simulink model "one_dim_sim"  (R2023a)
settings: Solver=VariableStepAuto  StartTime=0.0  StopTime=140  RelTol=1e-3
undefined symbols (not defined in the file): area_f, cd, g, mass, rho_m, volume
settings Model: Creator=erick  LastModifiedBy=erick

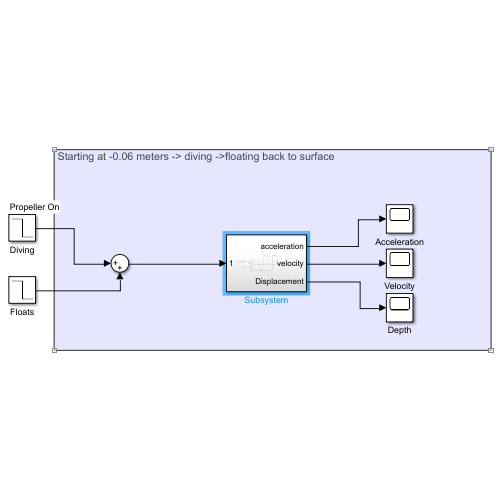
[thumbnail: Simulink's stored preview of the top-level diagram]
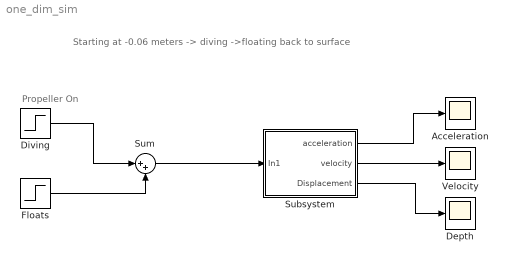
== system one_dim_sim ==
  note: Propeller On
  note: Starting at -0.06 meters -> diving ->floating back to surface
  Acceleration : Scope
  Depth : Scope
  Diving : Step  Time=60  Before=1.9  SampleTime=5
  Floats : Step  Time=80  After=-1  SampleTime=0
  Subsystem : Subsystem
  Sum : Sum  Inputs=|++
  Velocity : Scope
  wires:
  Subsystem/1(acceleration) -> Acceleration/1
  Subsystem/2(velocity) -> Velocity/1
  Subsystem/3(Displacement) -> Depth/1
  Diving/1 -> Sum/1
  Floats/1 -> Sum/2
  Sum/1 -> Subsystem/1(In1)

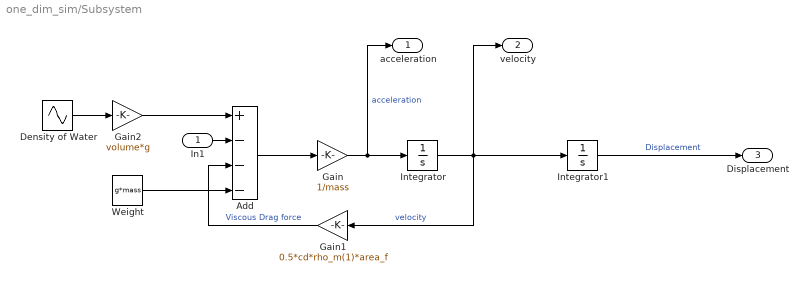
== system one_dim_sim/Subsystem ==
  In1 : Inport
  Add : Sum  Inputs=+---
  Density of Water : Sin  Amplitude=3  Bias=1000  Frequency=100  SampleTime=0
  Gain : Gain  Gain=1/mass
  Gain1 : Gain  Gain=0.5*cd*rho_m(1)*area_f
  Gain2 : Gain  Gain=volume*g
  Integrator : Integrator
  Integrator1 : Integrator  InitialCondition=-0.07
  Weight : Constant  Value=g*mass
  acceleration : Outport
  velocity : Outport  Port=2
  Displacement : Outport  Port=3
  wires:
  Add/1 -> Gain/1
  Integrator/1 -> velocity/1, Gain1/1, Integrator1/1  "velocity"
  Gain2/1 -> Add/1
  Weight/1 -> Add/4
  Gain/1 -> acceleration/1, Integrator/1  "acceleration"
  Gain1/1 -> Add/3  "Viscous Drag force"
  Integrator1/1 -> Displacement/1  "Displacement"
  In1/1 -> Add/2
  Density of Water/1 -> Gain2/1
